simulink model "phan_tich_he_thong_ode_r2021b"  (R2021b)
settings: Solver=FixedStepAuto  StartTime=0.0  StopTime=80  FixedStep=0.0001  RelTol=1e-3
undefined symbols (not defined in the file): B, b, g, L, m1, m2
settings Model: SimulationMode=accelerator  Creator=datng  LastModifiedBy=datng
settings DebuggingCC: UnconnectedInputMsg=none  UnconnectedOutputMsg=none  UnconnectedLineMsg=none
settings ModelReferenceCC: EnableRefExpFcnMdlSchedulingChecks=off
settings RTWCC: GPUComputeCapability=5.0  DLArmComputeVersion=20.02.1
settings ConfigComp: CovBoundaryAbsTol=1.0e-5

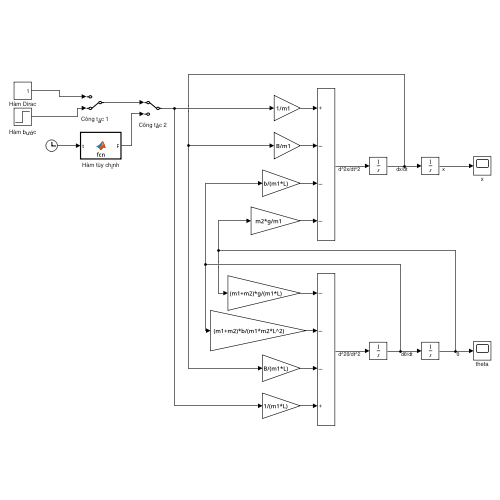
[thumbnail: Simulink's stored preview of the top-level diagram]
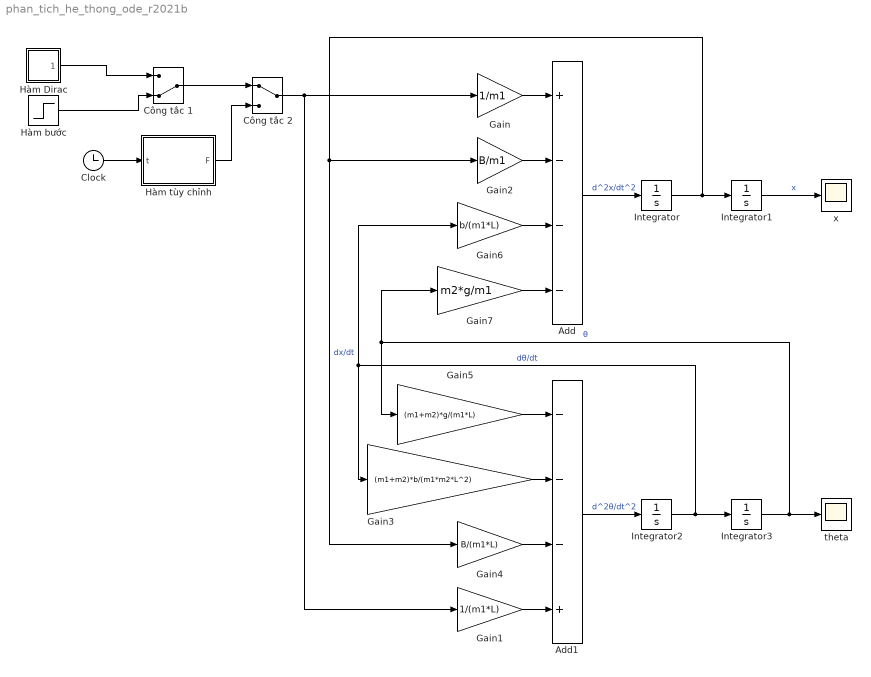
== system phan_tich_he_thong_ode_r2021b ==
  Add : Sum  Inputs=+---
  Add1 : Sum  Inputs=---+
  Clock : Clock
  Công tắc 1 : ManualSwitch  CurrentSetting=0
  Công tắc 2 : ManualSwitch
  Gain : Gain  Gain=1/m1
  Gain1 : Gain  Gain=1/(m1*L)
  Gain2 : Gain  Gain=B/m1
  Gain3 : Gain  Gain=(m1+m2)*b/(m1*m2*L^2)
  Gain4 : Gain  Gain=B/(m1*L)
  Gain5 : Gain  Gain=(m1+m2)*g/(m1*L)
  Gain6 : Gain  Gain=b/(m1*L)
  Gain7 : Gain  Gain=m2*g/m1
  Hàm Dirac : Subsystem
  Hàm bước : Step  Time=0  SampleTime=0
  Hàm tùy chỉnh : MATLAB Function  TreatAsAtomicUnit=on
  Integrator{,1..3} (4 alike) : Integrator
  theta : Scope
  x : Scope
  wires:
  Gain/1 -> Add/1
  Add/1 -> Integrator/1  "d^2x/dt^2"
  Integrator/1 -> Gain2/1, Gain4/1, Integrator1/1  "dx/dt"
  Gain2/1 -> Add/2
  Gain6/1 -> Add/3
  Gain7/1 -> Add/4
  Gain1/1 -> Add1/4
  Gain5/1 -> Add1/1
  Add1/1 -> Integrator2/1  "d^2θ/dt^2"
  Gain4/1 -> Add1/3
  Gain3/1 -> Add1/2
  Integrator2/1 -> Gain3/1, Gain6/1, Integrator3/1  "dθ/dt"
  Integrator3/1 -> theta/1, Gain5/1, Gain7/1  "θ"
  Hàm bước/1 -> Công tắc 1/2
  Clock/1 -> Hàm tùy chỉnh/1(t)
  Hàm tùy chỉnh/1(F) -> Công tắc 2/2
  Công tắc 1/1 -> Công tắc 2/1
  Công tắc 2/1 -> Gain1/1, Gain/1
  Integrator1/1 -> x/1  "x"
  Hàm Dirac/1(1) -> Công tắc 1/1

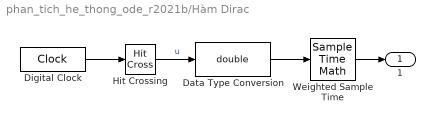
== system phan_tich_he_thong_ode_r2021b/Hàm Dirac ==
  Data Type Conversion : DataTypeConversion  OutDataTypeStr=double
  Digital Clock : DigitalClock  SampleTime=0.001
  Hit Crossing : HitCross
  Weighted Sample Time : SampleTimeMath  TsampMathOp=/
  1 : Outport
  wires:
  Digital Clock/1 -> Hit Crossing/1
  Hit Crossing/1 -> Data Type Conversion/1  "u"
  Data Type Conversion/1 -> Weighted Sample Time/1
  Weighted Sample Time/1 -> 1/1

== matlab function phan_tich_he_thong_ode_r2021b/Hàm tùy chỉnh ==
  data: t input; F output
function F = fcn(t)
    if t >= 0 && t <= 5
        F = 10;
    else
        F = 0;
    end
end
